simulink model "demo_interconnect"  (Simulink 7.4)
settings: Solver=ode45  StartTime=0.0  StopTime=100  RelTol=1e-3
undefined symbols (not defined in the file): ROACH
libraries: xbsIndex_r4 x135, xps_library x13, casper_library x12, isi_correlator_lib x10, dspsigops x8
settings Model: Creator=wjm  LastModifiedBy=wjm
settings OptimizationCC: InitFltsAndDblsToZero=on

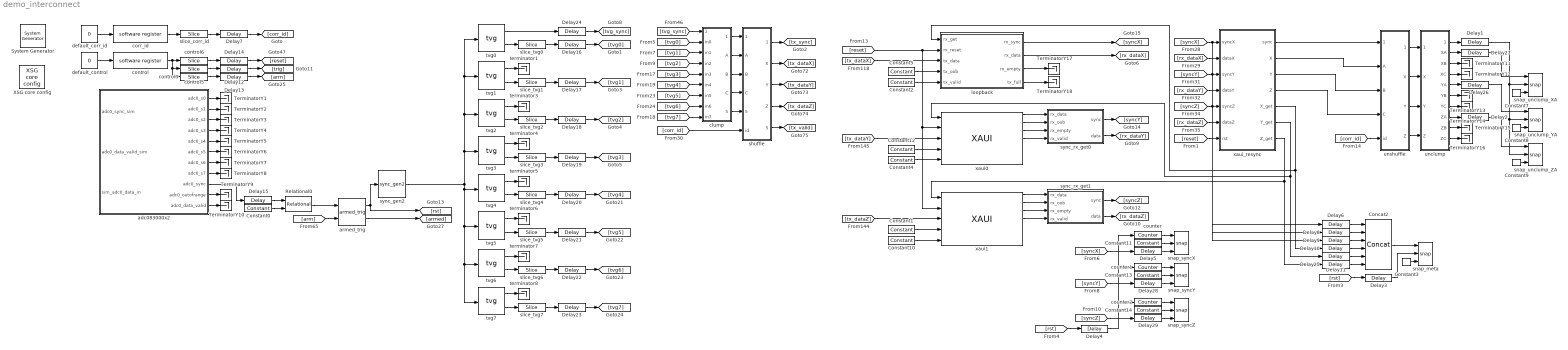
== system demo_interconnect ==
  " System Generator" : xbsIndex_r4/ System Generator  Tag=genX  SystemSampleTime=-1  xilinxfamily=virtex5  part=xc5vsx95t  speed=-1  package=ff1136  synthesis_tool=XST  clock_wrapper=Clock Enables  directory=./demo_interconnect/sysgen  testbench=off  simulink_period=1  sysclk_period=5  dcm_input_clock_period=100  incr_netlist=off  trim_vbits=Everywhere in SubSystem  dbl_ovrd=According to Block Masks  core_generation=According to Block Masks  run_coregen=off  deprecated_control=off  eval_field=0  block_type=sysgen
      settings: block_version=10.1.1
  Concat2 : xbsIndex_r4/Concat  num_inputs=6  dbl_ovrd=off  block_type=concat
      settings: block_version=11.3
  Constant{0..1,5,12} (4 alike) : xbsIndex_r4/Constant  arith_type=Unsigned  const=0  n_bits=4  bin_pt=0  explicit_period=on  period=1  equ=P=C  opselect=C  inp2=PCIN>>17  opr=+  inp1=P  carry=CIN  dbl_ovrd=off  block_type=constant
      Constant1 settings: block_version=10.1.1
      Constant12 settings: block_version=10.1.1
      Constant5 settings: block_version=10.1.1
  Constant{2..4,7..11,13..14} (10 alike) : xbsIndex_r4/Constant  arith_type=Boolean  const=1  n_bits=1  bin_pt=0  explicit_period=on  period=1  equ=P=C  opselect=C  inp2=PCIN>>17  opr=+  inp1=P  carry=CIN  dbl_ovrd=off  block_type=constant
      settings: block_version=10.1.1
  Delay{1..2,12..24,26..27} (17 alike) : xbsIndex_r4/Delay  en=off  latency=1  dbl_ovrd=off  reg_retiming=on  block_type=delay
  Delay{6,8..11,25} (6 alike) : xbsIndex_r4/Delay  en=off  latency=17  dbl_ovrd=off  reg_retiming=off  block_type=delay
  Delay{3..5,28..29} (5 alike) : xbsIndex_r4/Delay  en=off  latency=1  dbl_ovrd=off  reg_retiming=off  block_type=delay
  Delay7 : xbsIndex_r4/Delay  en=off  latency=0  dbl_ovrd=off  reg_retiming=on  block_type=delay
  Relational0 : xbsIndex_r4/Relational  mode=a!=b  en=off  latency=1  dbl_ovrd=off  block_type=relational
      settings: xl_area=[0, 0, 0, 0, 0, 0, 0]  block_version=10.1.3
  TerminatorY{1..18} (18 alike) : Terminator
  XSG core config : xps_library/XSG core config  Tag=xps:xsg  SystemSampleTime=-1  hw_sys=ROACH:sx95t  ibob_linux=off  clk_src=adc0_clk  iBOB_clk_src=sys_clk  BEE2_ctrl_clk_src=sys_clk  BEE2_usr_clk_src=sys_clk  ROACH_clk_src=adc0_clk  CORR_clk_src=sys_clk  gpio_clk_io_group=iBOB:sma  gpio_clk_bit_index=0  clk_rate=200  sample_period=1  synthesis_tool=XST  mpc_type=powerpc440_ext
  adc083000x2 : Subsystem  Tag=xps:adc083000x2  AncestorBlock=xps_library/adc083000x2  mask(adc_083000x2){use_adc0=on, use_adc1=off, demux_adc=off, clock_sync=off, verbose=off, using_ctrl=off, adc_clk_rate=800, sample_period=1, bit_width=8}
      mask prompts: use_adc0 "Use ZD0K0?"; use_adc1 "Use ZDOK1?"; demux_adc "Demux ADCs by 2?"; clock_sync "Interleave 2 ADC boards?"; verbose "Verbose Block Creation?"; using_ctrl "Add ports for control registers?"; adc_clk_rate "ADC clock rate (MHz)"; sample_period "Sample Period"; bit_width "Output Bit Width"
      mask help:
      | The ADC block converts analog inputs to digital outputs.
      | Every clock cycle, the inputs are sampled and digitized to
      | 8 bit binary point numbers in the range of [-1, 1).
      |
      | Online block-specific documentation: http://casper.berkeley.edu/wiki/Adc083000
      mask init:
      | adc083000_mask;
      mask Help: eval('xlWeb([getenv(''MLIB_ROOT''), ''\doc\html\sys_adc\sys_adc.html''])')
  armed_trig : isi_correlator_lib/armed_trig  SystemSampleTime=-1
  clump : Subsystem  AncestorBlock=isi_correlator_lib/clump  mask{latency=1}
  control : xps_library/software register  Tag=xps:sw_reg  SystemSampleTime=-1  io_dir=From Processor  arith_type=Unsigned  bitwidth=32  bin_pt=0  sample_period=1  gw_name=demo_interconnect_control_user_data_out
  control0 : xbsIndex_r4/Slice  nbits=1  boolean_output=on  mode=Lower Bit Location + Width  bit1=0  base1=MSB of Input  bit0=0  base0=LSB of Input  dbl_ovrd=off  block_type=slice
      settings: infoedit="Extracts a given range of bits from each input sample and presents it at the output.  The output type is ordinarily unsigned with binary point at zero, but can be Boolean when the slice is one bit wide.<P><P>Hardware notes: In hardware this block costs nothing."  block_version=10.1.3
  control5 : xbsIndex_r4/Slice  nbits=1  boolean_output=on  mode=Lower Bit Location + Width  bit1=0  base1=MSB of Input  bit0=1  base0=LSB of Input  dbl_ovrd=off  block_type=slice
      settings: infoedit="Extracts a given range of bits from each input sample and presents it at the output.  The output type is ordinarily unsigned with binary point at zero, but can be Boolean when the slice is one bit wide.<P><P>Hardware notes: In hardware this block costs nothing."  block_version=10.1.3
  control6 : xbsIndex_r4/Slice  nbits=1  boolean_output=on  mode=Lower Bit Location + Width  bit1=0  base1=MSB of Input  bit0=2  base0=LSB of Input  dbl_ovrd=off  block_type=slice
      settings: infoedit="Extracts a given range of bits from each input sample and presents it at the output.  The output type is ordinarily unsigned with binary point at zero, but can be Boolean when the slice is one bit wide.<P><P>Hardware notes: In hardware this block costs nothing."  block_version=10.1.3
  corr_id : xps_library/software register  Tag=xps:sw_reg  SystemSampleTime=-1  io_dir=From Processor  arith_type=Unsigned  bitwidth=32  bin_pt=0  sample_period=1  gw_name=demo_interconnect_corr_id_user_data_out
  counter : xbsIndex_r4/Counter  cnt_type=Free Running  cnt_to=Inf  operation=Up  start_count=0  cnt_by_val=1  arith_type=Unsigned  n_bits=32  bin_pt=0  load_pin=off  rst=on  en=off  explicit_period=on  period=1  dbl_ovrd=off  use_behavioral_HDL=off  implementation=Fabric  use_rpm=off  block_type=counter
  counter1 : xbsIndex_r4/Counter  cnt_type=Free Running  cnt_to=Inf  operation=Up  start_count=0  cnt_by_val=1  arith_type=Unsigned  n_bits=32  bin_pt=0  load_pin=off  rst=on  en=off  explicit_period=on  period=1  dbl_ovrd=off  use_behavioral_HDL=off  implementation=Fabric  use_rpm=off  block_type=counter
  counter2 : xbsIndex_r4/Counter  cnt_type=Free Running  cnt_to=Inf  operation=Up  start_count=0  cnt_by_val=1  arith_type=Unsigned  n_bits=32  bin_pt=0  load_pin=off  rst=on  en=off  explicit_period=on  period=1  dbl_ovrd=off  use_behavioral_HDL=off  implementation=Fabric  use_rpm=off  block_type=counter
  default_control : Constant  Value=0  OutDataType=sfix(16)  OutScaling=2^0  SampleTime=1
  default_corr_id : Constant  Value=0  OutDataType=sfix(16)  OutScaling=2^0  SampleTime=1
  loopback : Subsystem  AncestorBlock=isi_correlator_lib/loopback  mask(loopback){delay=8}
      mask prompts: delay "Delay: (2^?)"
      mask help:
      | A loopback link. Stores data in BRAM for long delay periods.
      |
      | Intended for buffering a stream of data until the other two
      | arrive over XAUI for resyncing.  Its delay should be set to
      | something on the order of (but less than) the XAUI latency.
  shuffle : Subsystem  AncestorBlock=isi_correlator_lib/shuffle  mask{latency=3}
  slice_corr_id : xbsIndex_r4/Slice  nbits=2  boolean_output=off  mode=Lower Bit Location + Width  bit1=0  base1=MSB of Input  bit0=0  base0=LSB of Input  dbl_ovrd=off  block_type=slice
      settings: infoedit="Extracts a given range of bits from each input sample and presents it at the output.  The output type is ordinarily unsigned with binary point at zero, but can be Boolean when the slice is one bit wide.<P><P>Hardware notes: In hardware this block costs nothing."  block_version=10.1.3
  slice_tvg{0..7} (8 alike) : xbsIndex_r4/Slice  nbits=8  boolean_output=off  mode=Lower Bit Location + Width  bit1=0  base1=MSB of Input  bit0=0  base0=LSB of Input  dbl_ovrd=off  block_type=slice
      settings: block_version=10.1.3
  snap_meta : casper_library/Scopes/snap  SystemSampleTime=-1  nsamples=13
  snap_syncX : casper_library/Scopes/snap  SystemSampleTime=-1  nsamples=13
  snap_syncY : casper_library/Scopes/snap  SystemSampleTime=-1  nsamples=13
  snap_syncZ : casper_library/Scopes/snap  SystemSampleTime=-1  nsamples=13
  snap_unclump_XA : casper_library/Scopes/snap  SystemSampleTime=-1  nsamples=13
  snap_unclump_YA : casper_library/Scopes/snap  SystemSampleTime=-1  nsamples=13
  snap_unclump_ZA : casper_library/Scopes/snap  SystemSampleTime=-1  nsamples=13
  sync_gen2 : isi_correlator_lib/sync_gen2  SystemSampleTime=-1
  sync_rx_get0 : Subsystem  AncestorBlock=isi_correlator_lib/sync_rx_get
  sync_rx_get1 : Subsystem  AncestorBlock=isi_correlator_lib/sync_rx_get
  terminator{1,3..8} (7 alike) : Terminator
  tvg{0..7} (8 alike) : isi_correlator_lib/tvg  SystemSampleTime=-1  addr_width=11
  unclump : Subsystem  AncestorBlock=isi_correlator_lib/unclump  mask{latency=1}
  unshuffle : Subsystem  AncestorBlock=isi_correlator_lib/unshuffle  mask{latency=3}
  xaui0 : xps_library/XAUI  Tag=xps:xaui  SystemSampleTime=-1  demux=2  port=ROACH:0  open_phy=off  show_param=off  pre_emph=3  swing=800
  xaui1 : xps_library/XAUI  Tag=xps:xaui  SystemSampleTime=-1  demux=2  port=ROACH:1  open_phy=off  show_param=off  pre_emph=3  swing=800
  xaui_resync : Subsystem  AncestorBlock=isi_correlator_lib/xaui_resync  mask(link_demux){buffer_depth=10, logic_latency=1}
      mask prompts: buffer_depth "Buffer depth: (2^?)"; logic_latency "Logic latency:"
      mask help:
      | Resynchronizes three data streams based on their sync pulses.
      |
      | Maximum buffer depth is 2^10.
  wires:
  armed_trig/1 -> sync_gen2/1, [rst]
  armed_trig/2 -> [armed]
  [tvg_sync] -> clump/1(sync)
  [tvg0] -> clump/2(in0)
  [tvg1] -> clump/3(in1)
  [tvg2] -> clump/4(in2)
  [tvg3] -> clump/5(in3)
  [tvg4] -> clump/6(in4)
  [tvg5] -> clump/7(in5)
  [tvg6] -> clump/8(in6)
  tvg0/2 -> slice_tvg0/1
  tvg1/2 -> slice_tvg1/1
  tvg2/2 -> slice_tvg2/1
  tvg0/1 -> Delay24/1
  tvg1/1 -> terminator1/1
  tvg2/1 -> terminator3/1
  tvg7/2 -> slice_tvg7/1
  tvg5/2 -> slice_tvg5/1
  tvg6/2 -> slice_tvg6/1
  tvg4/2 -> slice_tvg4/1
  tvg3/2 -> slice_tvg3/1
  tvg3/1 -> terminator4/1
  tvg4/1 -> terminator5/1
  tvg5/1 -> terminator6/1
  tvg6/1 -> terminator7/1
  tvg7/1 -> terminator8/1
  slice_tvg0/1 -> Delay16/1
  slice_tvg1/1 -> Delay17/1
  slice_tvg2/1 -> Delay18/1
  slice_tvg3/1 -> Delay19/1
  slice_tvg4/1 -> Delay20/1
  slice_tvg5/1 -> Delay21/1
  slice_tvg6/1 -> Delay22/1
  slice_tvg7/1 -> Delay23/1
  shuffle/1(sync_out) -> [tx_sync]
  shuffle/2(X) -> [tx_dataX]
  shuffle/3(Y) -> [tx_dataY]
  shuffle/4(Z) -> [tx_dataZ]
  shuffle/5(valid_out) -> [tx_valid]
  [tvg7] -> clump/9(in7)
  clump/1(sync_out) -> shuffle/1(sync)
  clump/2(A) -> shuffle/2(A)
  clump/3(B) -> shuffle/3(B)
  clump/4(C) -> shuffle/4(C)
  clump/5(valid) -> shuffle/5(valid)
  [corr_id] -> shuffle/6(id)
  unshuffle/1(sync_out) -> unclump/1(sync)
  unshuffle/2(X) -> unclump/2(X)
  unshuffle/3(Y) -> unclump/3(Y)
  unshuffle/4(Z) -> unclump/4(Z)
  [arm] -> armed_trig/2
  default_corr_id/1 -> corr_id/1
  corr_id/1 -> slice_corr_id/1
  Delay7/1 -> [corr_id]
  slice_corr_id/1 -> Delay7/1
  default_control/1 -> control/1
  control6/1 -> Delay14/1
  control5/1 -> Delay12/1
  control0/1 -> Delay13/1
  control/1 -> control6/1, control0/1, control5/1
  Delay14/1 -> [reset]
  Delay12/1 -> [trig]
  Delay13/1 -> [arm]
  adc083000x2/1(adc0_s0) -> TerminatorY1/1
  adc083000x2/2(adc0_s1) -> TerminatorY2/1
  adc083000x2/3(adc0_s2) -> TerminatorY3/1
  adc083000x2/4(adc0_s3) -> TerminatorY4/1
  adc083000x2/5(adc0_s4) -> TerminatorY5/1
  adc083000x2/6(adc0_s5) -> TerminatorY6/1
  adc083000x2/7(adc0_s6) -> TerminatorY7/1
  adc083000x2/8(adc0_s7) -> TerminatorY8/1
  adc083000x2/10(adc0_outofrange) -> TerminatorY9/1
  adc083000x2/11(adc0_data_valid) -> TerminatorY10/1
  Constant0/1 -> Relational0/2
  adc083000x2/9(adc0_sync) -> Delay15/1
  Delay15/1 -> Relational0/1
  Relational0/1 -> armed_trig/1
  sync_gen2/1 -> tvg4/1, tvg5/1, tvg7/1, tvg6/1, tvg3/1, tvg2/1, tvg0/1, tvg1/1
  Delay16/1 -> [tvg0]
  Delay17/1 -> [tvg1]
  Delay18/1 -> [tvg2]
  Delay19/1 -> [tvg3]
  Delay20/1 -> [tvg4]
  Delay21/1 -> [tvg5]
  Delay22/1 -> [tvg6]
  Delay23/1 -> [tvg7]
  Delay24/1 -> [tvg_sync]
  [tx_dataZ] -> xaui1/3
  Constant1/1 -> xaui1/4
  Constant12/1 -> xaui0/4
  [tx_dataY] -> xaui0/3
  Constant7/1 -> snap_unclump_XA/3
  Constant8/1 -> snap_unclump_YA/3
  Constant9/1 -> snap_unclump_ZA/3
  unclump/2(XA) -> Delay27/1
  unclump/5(YA) -> Delay26/1
  unclump/8(ZA) -> Delay2/1
  unclump/3(XB) -> TerminatorY11/1
  unclump/4(XC) -> TerminatorY12/1
  unclump/6(YB) -> TerminatorY13/1
  unclump/7(YC) -> TerminatorY14/1
  unclump/9(ZB) -> TerminatorY15/1
  unclump/10(ZC) -> TerminatorY16/1
  Delay2/1 -> snap_unclump_ZA/1
  Delay26/1 -> snap_unclump_YA/1
  Delay27/1 -> snap_unclump_XA/1
  xaui1/1 -> sync_rx_get1/1(rx_data)
  xaui1/2 -> sync_rx_get1/2(rx_oob)
  xaui1/3 -> sync_rx_get1/3(rx_empty)
  xaui1/4 -> sync_rx_get1/4(rx_valid)
  xaui0/1 -> sync_rx_get0/1(rx_data)
  xaui0/2 -> sync_rx_get0/2(rx_oob)
  xaui0/3 -> sync_rx_get0/3(rx_empty)
  xaui0/4 -> sync_rx_get0/4(rx_valid)
  [tx_dataX] -> loopback/3(tx_data)
  Constant2/1 -> loopback/5(tx_valid)
  Constant4/1 -> xaui0/5
  Constant10/1 -> xaui1/5
  [reset] -> loopback/2(rx_reset), xaui1/2, xaui0/2
  [corr_id] -> unshuffle/5(id)
  xaui_resync/1(sync) -> unshuffle/1(sync)
  xaui_resync/2(X) -> unshuffle/2(A)
  xaui_resync/3(Y) -> unshuffle/3(B)
  xaui_resync/4(Z) -> unshuffle/4(C)
  [syncX] -> xaui_resync/1(syncX), Delay6/1
  [rx_dataX] -> xaui_resync/2(dataX)
  [syncY] -> xaui_resync/3(syncY), Delay8/1
  [rx_dataY] -> xaui_resync/4(dataY)
  [syncZ] -> xaui_resync/5(syncZ), Delay9/1
  [rx_dataZ] -> xaui_resync/6(dataZ)
  xaui_resync/5(X_get) -> loopback/1(rx_get), Delay10/1
  xaui_resync/6(Y_get) -> xaui0/1, Delay11/1
  xaui_resync/7(Z_get) -> xaui1/1, Delay25/1
  [reset] -> xaui_resync/7(rst)
  loopback/1(rx_sync) -> [syncX]
  loopback/2(rx_data) -> [rx_dataX]
  Constant3/1 -> snap_meta/3
  Delay3/1 -> snap_meta/2
  [rst] -> Delay3/1
  Concat2/1 -> snap_meta/1
  sync_rx_get1/1(sync) -> [syncZ]
  sync_rx_get1/2(data) -> [rx_dataZ]
  sync_rx_get0/1(sync) -> [syncY]
  sync_rx_get0/2(data) -> [rx_dataY]
  Constant5/1 -> loopback/4(tx_oob)
  Delay6/1 -> Concat2/1
  Delay8/1 -> Concat2/2
  Delay9/1 -> Concat2/3
  Delay10/1 -> Concat2/4
  Delay11/1 -> Concat2/5
  Delay25/1 -> Concat2/6
  loopback/3(rx_empty) -> TerminatorY17/1
  loopback/4(tx_full) -> TerminatorY18/1
  Constant11/1 -> snap_syncX/2
  Constant13/1 -> snap_syncY/2
  Constant14/1 -> snap_syncZ/2
  [rst] -> Delay4/1
  counter/1 -> snap_syncX/1
  counter1/1 -> snap_syncY/1
  counter2/1 -> snap_syncZ/1
  Delay4/1 -> counter2/1, counter/1, counter1/1
  [syncX] -> Delay5/1
  [syncY] -> Delay28/1
  [syncZ] -> Delay29/1
  unclump/1(sync_out) -> Delay1/1
  Delay1/1 -> snap_unclump_XA/2, snap_unclump_ZA/2, snap_unclump_YA/2
  Delay5/1 -> snap_syncX/3
  Delay28/1 -> snap_syncY/3
  Delay29/1 -> snap_syncZ/3

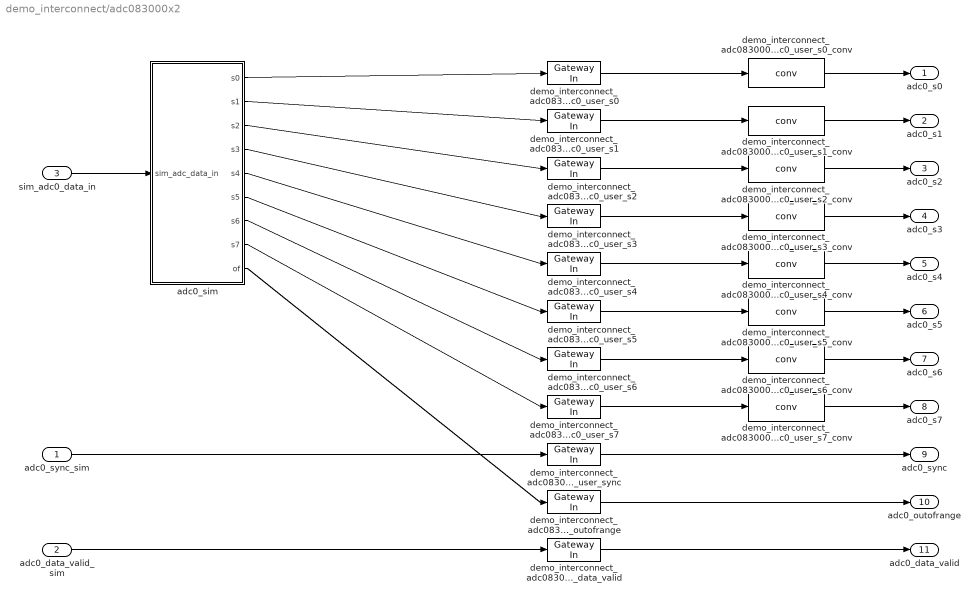
== system demo_interconnect/adc083000x2 ==
  adc0_sync_sim : Inport  OutDataType=sfix(16)  OutScaling=2^0
  adc0_data_valid_sim : Inport  Port=2  OutDataType=sfix(16)  OutScaling=2^0
  sim_adc0_data_in : Inport  Port=3  OutDataType=fixdt(1, 16)  OutScaling=2^0
  adc0_sim : Subsystem  AncestorBlock=xps_library/ADCs/adc_sim  mask(adc_sim){nStreams=8, bit_width=8}
      mask prompts: nStreams "Number of Output Streams"; bit_width "Sample Bit Width"
      mask help:
      | This block simulates the behavior of a demuxed ADC, which takes
      | as input a waveform and returns digital samples in parallel at
      | a slower rate.
      |
      | This block is used to simulate the behavior
      mask init:
      | adc_sim_init(gcb, ...
      |     'nStreams', nStreams, ...
      |     'bit_width', bit_width);
  demo_interconnect_adc083000x2_adc0_user_data_valid : xbsIndex_r4/Gateway In  arith_type=Unsigned  n_bits=1  bin_pt=0  quantization="Round  (unbiased: +/- Inf)"  overflow=Saturate  period=1  dbl_ovrd=off  timing_constraint=None  locs_specified=off  LOCs={}  hdl_port=on  block_type=gatewayin
      settings: infoedit="Gateway in block.  Converts inputs of type Simulink integer, double and fixed point to  Xilinx fixed point type.<br><br>Hardware notes:  In hardware these blocks become top level input ports."  block_version=11.4
  demo_interconnect_adc083000x2_adc0_user_outofrange : xbsIndex_r4/Gateway In  arith_type=Unsigned  n_bits=4  bin_pt=0  quantization="Round  (unbiased: +/- Inf)"  overflow=Saturate  period=1  dbl_ovrd=off  timing_constraint=None  locs_specified=off  LOCs={}  hdl_port=on  block_type=gatewayin
      settings: infoedit="Gateway in block.  Converts inputs of type Simulink integer, double and fixed point to  Xilinx fixed point type.<br><br>Hardware notes:  In hardware these blocks become top level input ports."  block_version=11.4
  demo_interconnect_adc083000x2_adc0_user_s{0..7} (8 alike) : xbsIndex_r4/Gateway In  arith_type=Unsigned  n_bits=8  bin_pt=0  quantization="Round  (unbiased: +/- Inf)"  overflow=Saturate  period=1  dbl_ovrd=off  timing_constraint=None  locs_specified=off  LOCs={}  hdl_port=on  block_type=gatewayin
      settings: infoedit="Gateway in block.  Converts inputs of type Simulink integer, double and fixed point to  Xilinx fixed point type.<br><br>Hardware notes:  In hardware these blocks become top level input ports."  block_version=11.4
  demo_interconnect_adc083000x2_adc0_user_s0_conv : xps_library/ADCs/conv  SystemSampleTime=-1  bit_width=8
  demo_interconnect_adc083000x2_adc0_user_s1_conv : xps_library/ADCs/conv  SystemSampleTime=-1  bit_width=8
  demo_interconnect_adc083000x2_adc0_user_s2_conv : xps_library/ADCs/conv  SystemSampleTime=-1  bit_width=8
  demo_interconnect_adc083000x2_adc0_user_s3_conv : xps_library/ADCs/conv  SystemSampleTime=-1  bit_width=8
  demo_interconnect_adc083000x2_adc0_user_s4_conv : xps_library/ADCs/conv  SystemSampleTime=-1  bit_width=8
  demo_interconnect_adc083000x2_adc0_user_s5_conv : xps_library/ADCs/conv  SystemSampleTime=-1  bit_width=8
  demo_interconnect_adc083000x2_adc0_user_s6_conv : xps_library/ADCs/conv  SystemSampleTime=-1  bit_width=8
  demo_interconnect_adc083000x2_adc0_user_s7_conv : xps_library/ADCs/conv  SystemSampleTime=-1  bit_width=8
  demo_interconnect_adc083000x2_adc0_user_sync : xbsIndex_r4/Gateway In  arith_type=Unsigned  n_bits=4  bin_pt=0  quantization="Round  (unbiased: +/- Inf)"  overflow=Saturate  period=1  dbl_ovrd=off  timing_constraint=None  locs_specified=off  LOCs={}  hdl_port=on  block_type=gatewayin
      settings: infoedit="Gateway in block.  Converts inputs of type Simulink integer, double and fixed point to  Xilinx fixed point type.<br><br>Hardware notes:  In hardware these blocks become top level input ports."  block_version=11.4
  adc0_s0 : Outport  OutDataType=fixdt(1, 16)  OutScaling=2^0
  adc0_s1 : Outport  Port=2  OutDataType=fixdt(1, 16)  OutScaling=2^0
  adc0_s2 : Outport  Port=3  OutDataType=fixdt(1, 16)  OutScaling=2^0
  adc0_s3 : Outport  Port=4  OutDataType=fixdt(1, 16)  OutScaling=2^0
  adc0_s4 : Outport  Port=5  OutDataType=fixdt(1, 16)  OutScaling=2^0
  adc0_s5 : Outport  Port=6  OutDataType=fixdt(1, 16)  OutScaling=2^0
  adc0_s6 : Outport  Port=7  OutDataType=fixdt(1, 16)  OutScaling=2^0
  adc0_s7 : Outport  Port=8  OutDataType=fixdt(1, 16)  OutScaling=2^0
  adc0_sync : Outport  Port=9  OutDataType=sfix(16)  OutScaling=2^0
  adc0_outofrange : Outport  Port=10  OutDataType=fixdt(1, 16)  OutScaling=2^0
  adc0_data_valid : Outport  Port=11  OutDataType=sfix(16)  OutScaling=2^0
  wires:
  sim_adc0_data_in/1 -> adc0_sim/1(sim_adc_data_in)
  adc0_sim/1(s0) -> demo_interconnect_adc083000x2_adc0_user_s0/1
  demo_interconnect_adc083000x2_adc0_user_s0/1 -> demo_interconnect_adc083000x2_adc0_user_s0_conv/1
  demo_interconnect_adc083000x2_adc0_user_s0_conv/1 -> adc0_s0/1
  adc0_sim/2(s1) -> demo_interconnect_adc083000x2_adc0_user_s1/1
  demo_interconnect_adc083000x2_adc0_user_s1/1 -> demo_interconnect_adc083000x2_adc0_user_s1_conv/1
  demo_interconnect_adc083000x2_adc0_user_s1_conv/1 -> adc0_s1/1
  adc0_sim/3(s2) -> demo_interconnect_adc083000x2_adc0_user_s2/1
  demo_interconnect_adc083000x2_adc0_user_s2/1 -> demo_interconnect_adc083000x2_adc0_user_s2_conv/1
  demo_interconnect_adc083000x2_adc0_user_s2_conv/1 -> adc0_s2/1
  adc0_sim/4(s3) -> demo_interconnect_adc083000x2_adc0_user_s3/1
  demo_interconnect_adc083000x2_adc0_user_s3/1 -> demo_interconnect_adc083000x2_adc0_user_s3_conv/1
  demo_interconnect_adc083000x2_adc0_user_s3_conv/1 -> adc0_s3/1
  adc0_sim/5(s4) -> demo_interconnect_adc083000x2_adc0_user_s4/1
  demo_interconnect_adc083000x2_adc0_user_s4/1 -> demo_interconnect_adc083000x2_adc0_user_s4_conv/1
  demo_interconnect_adc083000x2_adc0_user_s4_conv/1 -> adc0_s4/1
  adc0_sim/6(s5) -> demo_interconnect_adc083000x2_adc0_user_s5/1
  demo_interconnect_adc083000x2_adc0_user_s5/1 -> demo_interconnect_adc083000x2_adc0_user_s5_conv/1
  demo_interconnect_adc083000x2_adc0_user_s5_conv/1 -> adc0_s5/1
  adc0_sim/7(s6) -> demo_interconnect_adc083000x2_adc0_user_s6/1
  demo_interconnect_adc083000x2_adc0_user_s6/1 -> demo_interconnect_adc083000x2_adc0_user_s6_conv/1
  demo_interconnect_adc083000x2_adc0_user_s6_conv/1 -> adc0_s6/1
  adc0_sim/8(s7) -> demo_interconnect_adc083000x2_adc0_user_s7/1
  demo_interconnect_adc083000x2_adc0_user_s7/1 -> demo_interconnect_adc083000x2_adc0_user_s7_conv/1
  demo_interconnect_adc083000x2_adc0_user_s7_conv/1 -> adc0_s7/1
  adc0_sync_sim/1 -> demo_interconnect_adc083000x2_adc0_user_sync/1
  demo_interconnect_adc083000x2_adc0_user_sync/1 -> adc0_sync/1
  adc0_sim/9(of) -> demo_interconnect_adc083000x2_adc0_user_outofrange/1
  demo_interconnect_adc083000x2_adc0_user_outofrange/1 -> adc0_outofrange/1
  adc0_data_valid_sim/1 -> demo_interconnect_adc083000x2_adc0_user_data_valid/1
  demo_interconnect_adc083000x2_adc0_user_data_valid/1 -> adc0_data_valid/1

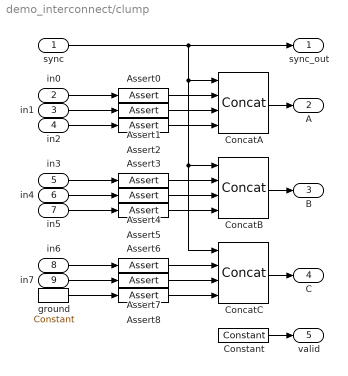
== system demo_interconnect/clump ==
  sync : Inport
  in0 : Inport  Port=2
  in1 : Inport  Port=3
  in2 : Inport  Port=4
  in3 : Inport  Port=5
  in4 : Inport  Port=6
  in5 : Inport  Port=7
  in6 : Inport  Port=8
  in7 : Inport  Port=9
  Assert{0..8} (9 alike) : xbsIndex_r4/Assert  assert_type=on  type_source=Explicitly  arith_type=Unsigned  n_bits=8  bin_pt=0  assert_rate=on  rate_source=Explicitly  period=1  output_port=on  block_type=assert
      settings: block_version=11.4
  ConcatA : xbsIndex_r4/Concat  num_inputs=4  dbl_ovrd=off  block_type=concat
      settings: block_version=11.3
  ConcatB : xbsIndex_r4/Concat  num_inputs=4  dbl_ovrd=off  block_type=concat
      settings: block_version=11.3
  ConcatC : xbsIndex_r4/Concat  num_inputs=4  dbl_ovrd=off  block_type=concat
      settings: block_version=11.3
  Constant : xbsIndex_r4/Constant  arith_type=Boolean  const=1  n_bits=1  bin_pt=0  explicit_period=on  period=1  equ=P=C  opselect=C  inp2=PCIN>>17  opr=+  inp1=P  carry=CIN  dbl_ovrd=off  block_type=constant
      settings: block_version=11.4
  ground : xbsIndex_r4/Constant  arith_type=Unsigned  const=0  n_bits=8  bin_pt=0  explicit_period=on  period=1  equ=P=C  opselect=C  inp2=PCIN>>17  opr=+  inp1=P  carry=CIN  dbl_ovrd=off  block_type=constant
      settings: block_version=10.1.1
  sync_out : Outport
  A : Outport  Port=2
  B : Outport  Port=3
  C : Outport  Port=4
  valid : Outport  Port=5
  wires:
  in2/1 -> Assert2/1
  in1/1 -> Assert1/1
  in0/1 -> Assert0/1
  ground/1 -> Assert8/1
  in7/1 -> Assert7/1
  in6/1 -> Assert6/1
  in5/1 -> Assert5/1
  in4/1 -> Assert4/1
  in3/1 -> Assert3/1
  sync/1 -> sync_out/1, ConcatA/1, ConcatC/1, ConcatB/1
  Constant/1 -> valid/1
  ConcatA/1 -> A/1
  ConcatB/1 -> B/1
  ConcatC/1 -> C/1
  Assert0/1 -> ConcatA/2
  Assert1/1 -> ConcatA/3
  Assert2/1 -> ConcatA/4
  Assert3/1 -> ConcatB/2
  Assert4/1 -> ConcatB/3
  Assert5/1 -> ConcatB/4
  Assert6/1 -> ConcatC/2
  Assert7/1 -> ConcatC/3
  Assert8/1 -> ConcatC/4

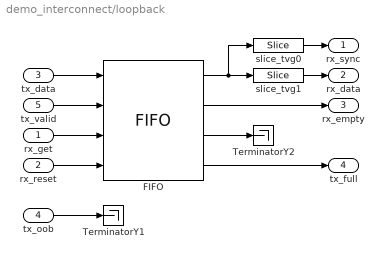
== system demo_interconnect/loopback ==
  rx_get : Inport  OutDataType=sfix(16)  OutScaling=2^0
  rx_reset : Inport  Port=2  OutDataType=sfix(16)  OutScaling=2^0
  tx_data : Inport  Port=3  OutDataType=sfix(16)  OutScaling=2^0
  tx_oob : Inport  Port=4  OutDataType=sfix(16)  OutScaling=2^0
  tx_valid : Inport  Port=5  OutDataType=sfix(16)  OutScaling=2^0
  FIFO : xbsIndex_r4/FIFO  depth=4K  percent_nbits=1  rst=on  en=off  use_dcount=off  use_almost_empty=off  almost_empty_thresh=2  use_almost_full=off  almost_full_thresh=14  dbl_ovrd=off  mem_type=Block RAM  explicit_period=off  block_type=fifo
      settings: block_version=11.4
  TerminatorY1 : Terminator
  TerminatorY2 : Terminator
  slice_tvg0 : xbsIndex_r4/Slice  nbits=1  boolean_output=on  mode=Lower Bit Location + Width  bit1=0  base1=MSB of Input  bit0=24  base0=LSB of Input  dbl_ovrd=off  block_type=slice
      settings: block_version=10.1.3
  slice_tvg1 : xbsIndex_r4/Slice  nbits=24  boolean_output=off  mode=Lower Bit Location + Width  bit1=0  base1=MSB of Input  bit0=0  base0=LSB of Input  dbl_ovrd=off  block_type=slice
      settings: block_version=10.1.3
  rx_sync : Outport  OutDataType=sfix(16)  OutScaling=2^0
  rx_data : Outport  Port=2  OutDataType=sfix(16)  OutScaling=2^0
  rx_empty : Outport  Port=3  OutDataType=sfix(16)  OutScaling=2^0
  tx_full : Outport  Port=4  OutDataType=sfix(16)  OutScaling=2^0
  wires:
  tx_data/1 -> FIFO/1
  tx_valid/1 -> FIFO/2
  rx_get/1 -> FIFO/3
  rx_reset/1 -> FIFO/4
  FIFO/2 -> rx_empty/1
  FIFO/1 -> slice_tvg1/1, slice_tvg0/1
  tx_oob/1 -> TerminatorY1/1
  slice_tvg1/1 -> rx_data/1
  slice_tvg0/1 -> rx_sync/1
  FIFO/4 -> tx_full/1
  FIFO/3 -> TerminatorY2/1

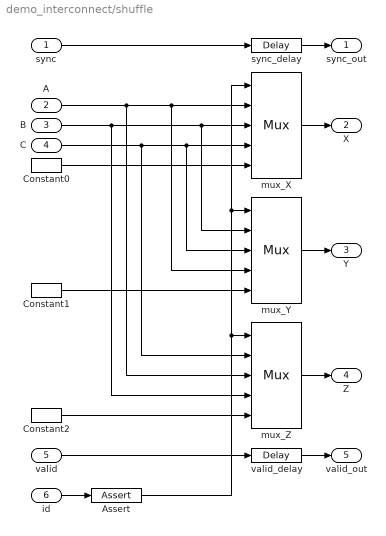
== system demo_interconnect/shuffle ==
  sync : Inport  OutDataType=sfix(16)  OutScaling=2^0
  A : Inport  Port=2  OutDataType=sfix(16)  OutScaling=2^0
  B : Inport  Port=3  OutDataType=sfix(16)  OutScaling=2^0
  C : Inport  Port=4  OutDataType=sfix(16)  OutScaling=2^0
  valid : Inport  Port=5  OutDataType=sfix(16)  OutScaling=2^0
  id : Inport  Port=6  OutDataType=sfix(16)  OutScaling=2^0
  Assert : xbsIndex_r4/Assert  assert_type=on  type_source=Explicitly  arith_type=Unsigned  n_bits=2  bin_pt=0  assert_rate=on  rate_source=Explicitly  period=1  output_port=on  block_type=assert
      settings: block_version=11.4
  Constant0 : xbsIndex_r4/Constant  arith_type=Unsigned  const=0  n_bits=25  bin_pt=0  explicit_period=on  period=1  equ=P=C  opselect=C  inp2=PCIN>>17  opr=+  inp1=P  carry=CIN  dbl_ovrd=off  block_type=constant
      settings: block_version=10.1.1
  Constant1 : xbsIndex_r4/Constant  arith_type=Unsigned  const=0  n_bits=25  bin_pt=0  explicit_period=on  period=1  equ=P=C  opselect=C  inp2=PCIN>>17  opr=+  inp1=P  carry=CIN  dbl_ovrd=off  block_type=constant
      settings: block_version=10.1.1
  Constant2 : xbsIndex_r4/Constant  arith_type=Unsigned  const=0  n_bits=25  bin_pt=0  explicit_period=on  period=1  equ=P=C  opselect=C  inp2=PCIN>>17  opr=+  inp1=P  carry=CIN  dbl_ovrd=off  block_type=constant
      settings: block_version=10.1.1
  mux_X : xbsIndex_r4/Mux  inputs=4  en=off  latency=latency  precision=Full  arith_type=Unsigned  n_bits=16  bin_pt=14  quantization=Truncate  overflow=Wrap  dbl_ovrd=off  block_type=mux
  mux_Y : xbsIndex_r4/Mux  inputs=4  en=off  latency=latency  precision=Full  arith_type=Unsigned  n_bits=16  bin_pt=14  quantization=Truncate  overflow=Wrap  dbl_ovrd=off  block_type=mux
  mux_Z : xbsIndex_r4/Mux  inputs=4  en=off  latency=latency  precision=Full  arith_type=Unsigned  n_bits=16  bin_pt=14  quantization=Truncate  overflow=Wrap  dbl_ovrd=off  block_type=mux
  sync_delay : xbsIndex_r4/Delay  en=off  latency=latency  dbl_ovrd=off  reg_retiming=off  block_type=delay
  valid_delay : xbsIndex_r4/Delay  en=off  latency=latency  dbl_ovrd=off  reg_retiming=off  block_type=delay
  sync_out : Outport  OutDataType=sfix(16)  OutScaling=2^0
  X : Outport  Port=2  OutDataType=sfix(16)  OutScaling=2^0
  Y : Outport  Port=3  OutDataType=sfix(16)  OutScaling=2^0
  Z : Outport  Port=4  OutDataType=sfix(16)  OutScaling=2^0
  valid_out : Outport  Port=5  OutDataType=sfix(16)  OutScaling=2^0
  wires:
  valid_delay/1 -> valid_out/1
  valid/1 -> valid_delay/1
  Assert/1 -> mux_Z/1, mux_Y/1, mux_X/1
  mux_Z/1 -> Z/1
  sync_delay/1 -> sync_out/1
  id/1 -> Assert/1
  sync/1 -> sync_delay/1
  C/1 -> mux_Z/2, mux_Y/3, mux_X/4
  B/1 -> mux_Z/4, mux_Y/2, mux_X/3
  A/1 -> mux_Z/3, mux_Y/4, mux_X/2
  mux_Y/1 -> Y/1
  mux_X/1 -> X/1
  Constant0/1 -> mux_X/5
  Constant1/1 -> mux_Y/5
  Constant2/1 -> mux_Z/5

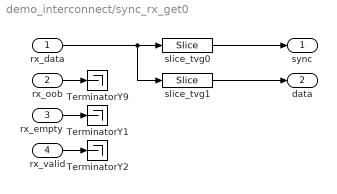
== system demo_interconnect/sync_rx_get0 ==
  rx_data : Inport
  rx_oob : Inport  Port=2
  rx_empty : Inport  Port=3
  rx_valid : Inport  Port=4
  TerminatorY1 : Terminator
  TerminatorY2 : Terminator
  TerminatorY9 : Terminator
  slice_tvg0 : xbsIndex_r4/Slice  nbits=1  boolean_output=on  mode=Lower Bit Location + Width  bit1=0  base1=MSB of Input  bit0=24  base0=LSB of Input  dbl_ovrd=off  block_type=slice
      settings: block_version=10.1.3
  slice_tvg1 : xbsIndex_r4/Slice  nbits=24  boolean_output=off  mode=Lower Bit Location + Width  bit1=0  base1=MSB of Input  bit0=0  base0=LSB of Input  dbl_ovrd=off  block_type=slice
      settings: block_version=10.1.3
  sync : Outport
  data : Outport  Port=2
  wires:
  rx_data/1 -> slice_tvg0/1, slice_tvg1/1
  slice_tvg0/1 -> sync/1
  slice_tvg1/1 -> data/1
  rx_oob/1 -> TerminatorY9/1
  rx_empty/1 -> TerminatorY1/1
  rx_valid/1 -> TerminatorY2/1

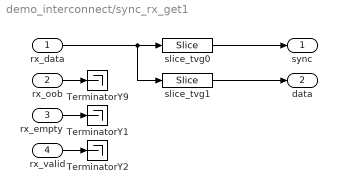
== system demo_interconnect/sync_rx_get1 ==
  rx_data : Inport
  rx_oob : Inport  Port=2
  rx_empty : Inport  Port=3
  rx_valid : Inport  Port=4
  TerminatorY1 : Terminator
  TerminatorY2 : Terminator
  TerminatorY9 : Terminator
  slice_tvg0 : xbsIndex_r4/Slice  nbits=1  boolean_output=on  mode=Lower Bit Location + Width  bit1=0  base1=MSB of Input  bit0=24  base0=LSB of Input  dbl_ovrd=off  block_type=slice
      settings: block_version=10.1.3
  slice_tvg1 : xbsIndex_r4/Slice  nbits=24  boolean_output=off  mode=Lower Bit Location + Width  bit1=0  base1=MSB of Input  bit0=0  base0=LSB of Input  dbl_ovrd=off  block_type=slice
      settings: block_version=10.1.3
  sync : Outport
  data : Outport  Port=2
  wires:
  rx_valid/1 -> TerminatorY2/1
  rx_empty/1 -> TerminatorY1/1
  rx_oob/1 -> TerminatorY9/1
  slice_tvg1/1 -> data/1
  slice_tvg0/1 -> sync/1
  rx_data/1 -> slice_tvg1/1, slice_tvg0/1

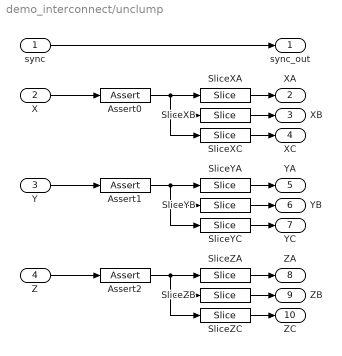
== system demo_interconnect/unclump ==
  sync : Inport
  X : Inport  Port=2
  Y : Inport  Port=3
  Z : Inport  Port=4
  Assert0 : xbsIndex_r4/Assert  assert_type=on  type_source=Explicitly  arith_type=Unsigned  n_bits=24  bin_pt=0  assert_rate=on  rate_source=Explicitly  period=1  output_port=on  block_type=assert
      settings: block_version=11.4
  Assert1 : xbsIndex_r4/Assert  assert_type=on  type_source=Explicitly  arith_type=Unsigned  n_bits=24  bin_pt=0  assert_rate=on  rate_source=Explicitly  period=1  output_port=on  block_type=assert
      settings: block_version=11.4
  Assert2 : xbsIndex_r4/Assert  assert_type=on  type_source=Explicitly  arith_type=Unsigned  n_bits=24  bin_pt=0  assert_rate=on  rate_source=Explicitly  period=1  output_port=on  block_type=assert
      settings: block_version=11.4
  SliceXA : xbsIndex_r4/Slice  nbits=8  boolean_output=off  mode=Lower Bit Location + Width  bit1=0  base1=MSB of Input  bit0=16  base0=LSB of Input  dbl_ovrd=off  block_type=slice
      settings: block_version=10.1.1
  SliceXB : xbsIndex_r4/Slice  nbits=8  boolean_output=off  mode=Lower Bit Location + Width  bit1=0  base1=MSB of Input  bit0=8  base0=LSB of Input  dbl_ovrd=off  block_type=slice
      settings: block_version=10.1.1
  SliceXC : xbsIndex_r4/Slice  nbits=8  boolean_output=off  mode=Lower Bit Location + Width  bit1=0  base1=MSB of Input  bit0=0  base0=LSB of Input  dbl_ovrd=off  block_type=slice
      settings: block_version=10.1.1
  SliceYA : xbsIndex_r4/Slice  nbits=8  boolean_output=off  mode=Lower Bit Location + Width  bit1=0  base1=MSB of Input  bit0=16  base0=LSB of Input  dbl_ovrd=off  block_type=slice
      settings: block_version=10.1.1
  SliceYB : xbsIndex_r4/Slice  nbits=8  boolean_output=off  mode=Lower Bit Location + Width  bit1=0  base1=MSB of Input  bit0=8  base0=LSB of Input  dbl_ovrd=off  block_type=slice
      settings: block_version=10.1.1
  SliceYC : xbsIndex_r4/Slice  nbits=8  boolean_output=off  mode=Lower Bit Location + Width  bit1=0  base1=MSB of Input  bit0=0  base0=LSB of Input  dbl_ovrd=off  block_type=slice
      settings: block_version=10.1.1
  SliceZA : xbsIndex_r4/Slice  nbits=8  boolean_output=off  mode=Lower Bit Location + Width  bit1=0  base1=MSB of Input  bit0=16  base0=LSB of Input  dbl_ovrd=off  block_type=slice
      settings: block_version=10.1.1
  SliceZB : xbsIndex_r4/Slice  nbits=8  boolean_output=off  mode=Lower Bit Location + Width  bit1=0  base1=MSB of Input  bit0=8  base0=LSB of Input  dbl_ovrd=off  block_type=slice
      settings: block_version=10.1.1
  SliceZC : xbsIndex_r4/Slice  nbits=8  boolean_output=off  mode=Lower Bit Location + Width  bit1=0  base1=MSB of Input  bit0=0  base0=LSB of Input  dbl_ovrd=off  block_type=slice
      settings: block_version=10.1.1
  sync_out : Outport
  XA : Outport  Port=2
  XB : Outport  Port=3
  XC : Outport  Port=4
  YA : Outport  Port=5
  YB : Outport  Port=6
  YC : Outport  Port=7
  ZA : Outport  Port=8
  ZB : Outport  Port=9
  ZC : Outport  Port=10
  wires:
  sync/1 -> sync_out/1
  X/1 -> Assert0/1
  Y/1 -> Assert1/1
  Z/1 -> Assert2/1
  Assert0/1 -> SliceXA/1, SliceXC/1, SliceXB/1
  Assert1/1 -> SliceYA/1, SliceYC/1, SliceYB/1
  Assert2/1 -> SliceZA/1, SliceZC/1, SliceZB/1
  SliceXA/1 -> XA/1
  SliceXB/1 -> XB/1
  SliceXC/1 -> XC/1
  SliceYA/1 -> YA/1
  SliceYB/1 -> YB/1
  SliceYC/1 -> YC/1
  SliceZA/1 -> ZA/1
  SliceZB/1 -> ZB/1
  SliceZC/1 -> ZC/1

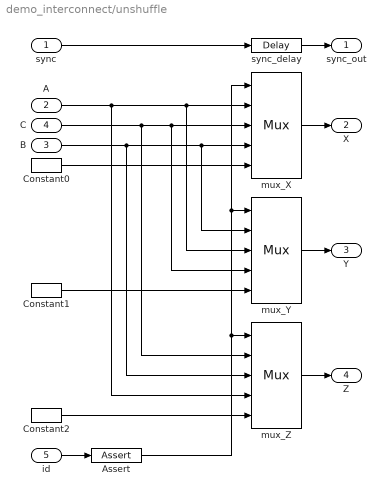
== system demo_interconnect/unshuffle ==
  sync : Inport  OutDataType=sfix(16)  OutScaling=2^0
  A : Inport  Port=2  OutDataType=sfix(16)  OutScaling=2^0
  B : Inport  Port=3  OutDataType=sfix(16)  OutScaling=2^0
  C : Inport  Port=4  OutDataType=sfix(16)  OutScaling=2^0
  id : Inport  Port=5  OutDataType=sfix(16)  OutScaling=2^0
  Assert : xbsIndex_r4/Assert  assert_type=on  type_source=Explicitly  arith_type=Unsigned  n_bits=2  bin_pt=0  assert_rate=on  rate_source=Explicitly  period=1  output_port=on  block_type=assert
      settings: block_version=11.4
  Constant0 : xbsIndex_r4/Constant  arith_type=Unsigned  const=0  n_bits=24  bin_pt=0  explicit_period=on  period=1  equ=P=C  opselect=C  inp2=PCIN>>17  opr=+  inp1=P  carry=CIN  dbl_ovrd=off  block_type=constant
      settings: block_version=10.1.1
  Constant1 : xbsIndex_r4/Constant  arith_type=Unsigned  const=0  n_bits=24  bin_pt=0  explicit_period=on  period=1  equ=P=C  opselect=C  inp2=PCIN>>17  opr=+  inp1=P  carry=CIN  dbl_ovrd=off  block_type=constant
      settings: block_version=10.1.1
  Constant2 : xbsIndex_r4/Constant  arith_type=Unsigned  const=0  n_bits=24  bin_pt=0  explicit_period=on  period=1  equ=P=C  opselect=C  inp2=PCIN>>17  opr=+  inp1=P  carry=CIN  dbl_ovrd=off  block_type=constant
      settings: block_version=10.1.1
  mux_X : xbsIndex_r4/Mux  inputs=4  en=off  latency=latency  precision=Full  arith_type=Unsigned  n_bits=16  bin_pt=14  quantization=Truncate  overflow=Wrap  dbl_ovrd=off  block_type=mux
  mux_Y : xbsIndex_r4/Mux  inputs=4  en=off  latency=latency  precision=Full  arith_type=Unsigned  n_bits=16  bin_pt=14  quantization=Truncate  overflow=Wrap  dbl_ovrd=off  block_type=mux
  mux_Z : xbsIndex_r4/Mux  inputs=4  en=off  latency=latency  precision=Full  arith_type=Unsigned  n_bits=16  bin_pt=14  quantization=Truncate  overflow=Wrap  dbl_ovrd=off  block_type=mux
  sync_delay : xbsIndex_r4/Delay  en=off  latency=latency  dbl_ovrd=off  reg_retiming=off  block_type=delay
  sync_out : Outport  OutDataType=sfix(16)  OutScaling=2^0
  X : Outport  Port=2  OutDataType=sfix(16)  OutScaling=2^0
  Y : Outport  Port=3  OutDataType=sfix(16)  OutScaling=2^0
  Z : Outport  Port=4  OutDataType=sfix(16)  OutScaling=2^0
  wires:
  Constant2/1 -> mux_Z/5
  Constant1/1 -> mux_Y/5
  Constant0/1 -> mux_X/5
  mux_X/1 -> X/1
  mux_Y/1 -> Y/1
  A/1 -> mux_Z/4, mux_X/2, mux_Y/3
  C/1 -> mux_X/3, mux_Y/4, mux_Z/2
  B/1 -> mux_X/4, mux_Y/2, mux_Z/3
  sync/1 -> sync_delay/1
  id/1 -> Assert/1
  sync_delay/1 -> sync_out/1
  mux_Z/1 -> Z/1
  Assert/1 -> mux_X/1, mux_Y/1, mux_Z/1

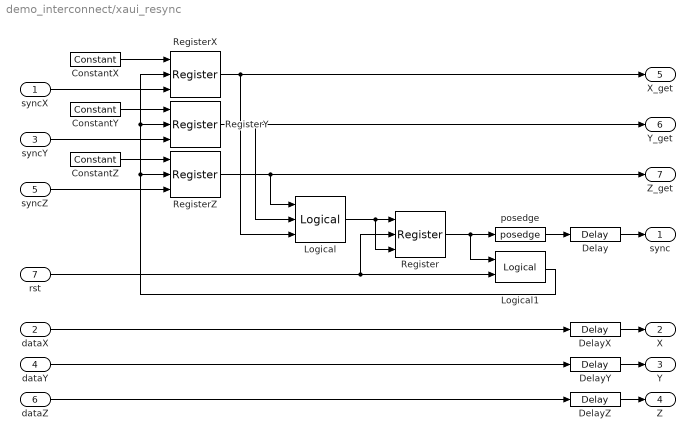
== system demo_interconnect/xaui_resync ==
  syncX : Inport  OutDataType=sfix(16)  OutScaling=2^0
  dataX : Inport  Port=2  OutDataType=sfix(16)  OutScaling=2^0
  syncY : Inport  Port=3  OutDataType=sfix(16)  OutScaling=2^0
  dataY : Inport  Port=4  OutDataType=sfix(16)  OutScaling=2^0
  syncZ : Inport  Port=5  OutDataType=sfix(16)  OutScaling=2^0
  dataZ : Inport  Port=6  OutDataType=sfix(16)  OutScaling=2^0
  rst : Inport  Port=7  OutDataType=sfix(16)  OutScaling=2^0
  ConstantX : xbsIndex_r4/Constant  arith_type=Boolean  const=0  n_bits=1  bin_pt=0  explicit_period=on  period=1  equ=P=C  opselect=C  inp2=PCIN>>17  opr=+  inp1=P  carry=CIN  dbl_ovrd=off  block_type=constant
      settings: block_version=10.1.1
  ConstantY : xbsIndex_r4/Constant  arith_type=Boolean  const=0  n_bits=1  bin_pt=0  explicit_period=on  period=1  equ=P=C  opselect=C  inp2=PCIN>>17  opr=+  inp1=P  carry=CIN  dbl_ovrd=off  block_type=constant
      settings: block_version=10.1.1
  ConstantZ : xbsIndex_r4/Constant  arith_type=Boolean  const=0  n_bits=1  bin_pt=0  explicit_period=on  period=1  equ=P=C  opselect=C  inp2=PCIN>>17  opr=+  inp1=P  carry=CIN  dbl_ovrd=off  block_type=constant
      settings: block_version=10.1.1
  Delay : xbsIndex_r4/Delay  en=off  latency=1  dbl_ovrd=off  reg_retiming=on  block_type=delay
  DelayX : xbsIndex_r4/Delay  en=off  latency=1  dbl_ovrd=off  reg_retiming=on  block_type=delay
  DelayY : xbsIndex_r4/Delay  en=off  latency=logic_latency  dbl_ovrd=off  reg_retiming=on  block_type=delay
  DelayZ : xbsIndex_r4/Delay  en=off  latency=logic_latency  dbl_ovrd=off  reg_retiming=on  block_type=delay
  Logical : xbsIndex_r4/Logical  logical_function=NOR  inputs=3  en=off  latency=1  precision=Full  arith_type=Unsigned  n_bits=16  bin_pt=0  align_bp=on  dbl_ovrd=off  block_type=logical
      settings: block_version=11.4
  Logical1 : xbsIndex_r4/Logical  logical_function=OR  inputs=2  en=off  latency=0  precision=Full  arith_type=Unsigned  n_bits=16  bin_pt=0  align_bp=on  dbl_ovrd=off  block_type=logical
      settings: block_version=11.4
  Register : xbsIndex_r4/Register  init=0  rst=on  en=on  dbl_ovrd=off  block_type=register
      settings: block_version=11.4
  RegisterX : xbsIndex_r4/Register  init=1  rst=on  en=on  dbl_ovrd=off  block_type=register
      settings: block_version=11.4
  RegisterY : xbsIndex_r4/Register  init=1  rst=on  en=on  dbl_ovrd=off  block_type=register
      settings: block_version=11.4
  RegisterZ : xbsIndex_r4/Register  init=1  rst=on  en=on  dbl_ovrd=off  block_type=register
      settings: block_version=11.4
  posedge : casper_library/Misc/posedge  Tag=Rising Edge Detector  SystemSampleTime=-1
  sync : Outport  OutDataType=sfix(16)  OutScaling=2^0
  X : Outport  Port=2  OutDataType=sfix(16)  OutScaling=2^0
  Y : Outport  Port=3  OutDataType=sfix(16)  OutScaling=2^0
  Z : Outport  Port=4  OutDataType=sfix(16)  OutScaling=2^0
  X_get : Outport  Port=5  OutDataType=sfix(16)  OutScaling=2^0
  Y_get : Outport  Port=6  OutDataType=sfix(16)  OutScaling=2^0
  Z_get : Outport  Port=7  OutDataType=sfix(16)  OutScaling=2^0
  wires:
  DelayZ/1 -> Z/1
  DelayY/1 -> Y/1
  ConstantX/1 -> RegisterX/1
  ConstantY/1 -> RegisterY/1
  ConstantZ/1 -> RegisterZ/1
  syncX/1 -> RegisterX/3
  syncY/1 -> RegisterY/3
  syncZ/1 -> RegisterZ/3
  DelayX/1 -> X/1
  dataX/1 -> DelayX/1
  dataY/1 -> DelayY/1
  dataZ/1 -> DelayZ/1
  RegisterY/1 -> Y_get/1, Logical/2
  RegisterX/1 -> X_get/1, Logical/3
  RegisterZ/1 -> Z_get/1, Logical/1
  Logical/1 -> Register/1, Register/3
  posedge/1 -> Delay/1
  Delay/1 -> sync/1
  Register/1 -> Logical1/1, posedge/1
  rst/1 -> Logical1/2, Register/2
  Logical1/1 -> RegisterX/2, RegisterY/2, RegisterZ/2

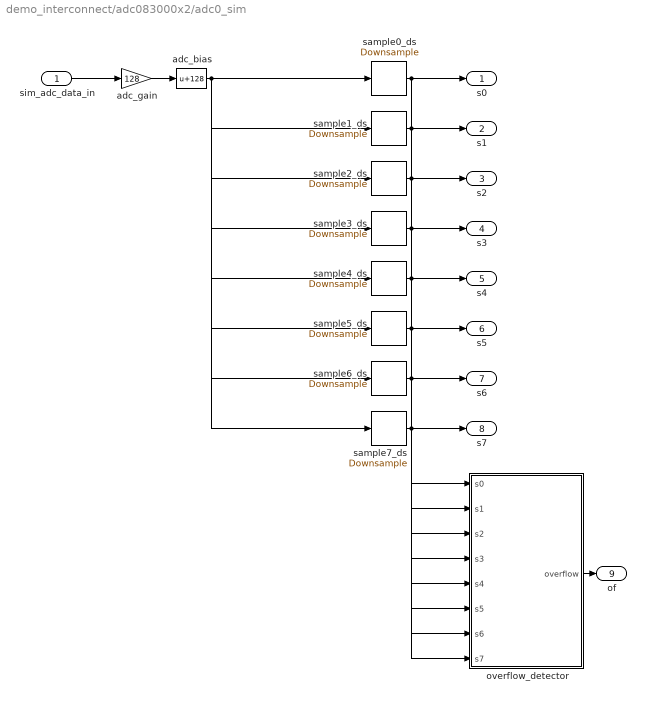
== system demo_interconnect/adc083000x2/adc0_sim ==
  sim_adc_data_in : Inport  OutDataType=sfix(16)  OutScaling=2^0
  adc_bias : Bias  Bias=128  SaturateOnIntegerOverflow=on
  adc_gain : Gain  Gain=128  ParameterDataType=sfix(16)  ParameterScaling=2^0  OutDataType=sfix(16)  OutScaling=2^0
  overflow_detector : Subsystem  AncestorBlock=casper_library/Misc/of_detect_bus  mask(of_detect_bus){nStreams=8, bit_width=8}
      mask prompts: nStreams "Number of Streams"; bit_width "Bit Width"
      mask init:
      | adc_overflow_detector_init(gcb, ...
      |     'nStreams', nStreams, ...
      |     'bit_width', bit_width);
  sample0_ds : dspsigops/Downsample  N=8  phase=1  ic=0  smode=Force single rate  fmode=Maintain input frame size
  sample1_ds : dspsigops/Downsample  N=8  phase=2  ic=0  smode=Force single rate  fmode=Maintain input frame size
  sample2_ds : dspsigops/Downsample  N=8  phase=3  ic=0  smode=Force single rate  fmode=Maintain input frame size
  sample3_ds : dspsigops/Downsample  N=8  phase=4  ic=0  smode=Force single rate  fmode=Maintain input frame size
  sample4_ds : dspsigops/Downsample  N=8  phase=5  ic=0  smode=Force single rate  fmode=Maintain input frame size
  sample5_ds : dspsigops/Downsample  N=8  phase=6  ic=0  smode=Force single rate  fmode=Maintain input frame size
  sample6_ds : dspsigops/Downsample  N=8  phase=7  ic=0  smode=Force single rate  fmode=Maintain input frame size
  sample7_ds : dspsigops/Downsample  N=8  phase=0  ic=0  smode=Force single rate  fmode=Maintain input frame size
  s0 : Outport  OutDataType=sfix(16)  OutScaling=2^0
  s1 : Outport  Port=2  OutDataType=sfix(16)  OutScaling=2^0
  s2 : Outport  Port=3  OutDataType=sfix(16)  OutScaling=2^0
  s3 : Outport  Port=4  OutDataType=sfix(16)  OutScaling=2^0
  s4 : Outport  Port=5  OutDataType=sfix(16)  OutScaling=2^0
  s5 : Outport  Port=6  OutDataType=sfix(16)  OutScaling=2^0
  s6 : Outport  Port=7  OutDataType=sfix(16)  OutScaling=2^0
  s7 : Outport  Port=8  OutDataType=sfix(16)  OutScaling=2^0
  of : Outport  Port=9  OutDataType=sfix(16)  OutScaling=2^0
  wires:
  sim_adc_data_in/1 -> adc_gain/1
  adc_gain/1 -> adc_bias/1
  overflow_detector/1(overflow) -> of/1
  adc_bias/1 -> sample0_ds/1, sample1_ds/1, sample2_ds/1, sample3_ds/1, sample4_ds/1, sample5_ds/1, sample6_ds/1, sample7_ds/1
  sample0_ds/1 -> overflow_detector/1(s0), s0/1
  sample1_ds/1 -> overflow_detector/2(s1), s1/1
  sample2_ds/1 -> overflow_detector/3(s2), s2/1
  sample3_ds/1 -> overflow_detector/4(s3), s3/1
  sample4_ds/1 -> overflow_detector/5(s4), s4/1
  sample5_ds/1 -> overflow_detector/6(s5), s5/1
  sample6_ds/1 -> overflow_detector/7(s6), s6/1
  sample7_ds/1 -> overflow_detector/8(s7), s7/1

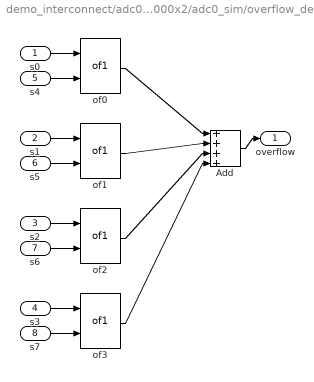
== system demo_interconnect/adc083000x2/adc0_sim/overflow_detector ==
  s0 : Inport  OutDataType=fixdt(1, 16)  OutScaling=2^0
  s1 : Inport  Port=2  OutDataType=fixdt(1, 16)  OutScaling=2^0
  s2 : Inport  Port=3  OutDataType=fixdt(1, 16)  OutScaling=2^0
  s3 : Inport  Port=4  OutDataType=fixdt(1, 16)  OutScaling=2^0
  s4 : Inport  Port=5  OutDataType=fixdt(1, 16)  OutScaling=2^0
  s5 : Inport  Port=6  OutDataType=fixdt(1, 16)  OutScaling=2^0
  s6 : Inport  Port=7  OutDataType=fixdt(1, 16)  OutScaling=2^0
  s7 : Inport  Port=8  OutDataType=fixdt(1, 16)  OutScaling=2^0
  Add : Sum  Inputs=++++  OutDataType=fixdt(1, 16)  OutScaling=2^-10
  of{0..3} (4 alike) : casper_library/Misc/of1  SystemSampleTime=-1  bit_num=0  n_adc_bits=8
  overflow : Outport  OutDataType=fixdt(1, 16)  OutScaling=2^0
  wires:
  s0/1 -> of0/1
  s4/1 -> of0/2
  of0/1 -> Add/1
  s1/1 -> of1/1
  s5/1 -> of1/2
  of1/1 -> Add/2
  s2/1 -> of2/1
  s6/1 -> of2/2
  of2/1 -> Add/3
  s3/1 -> of3/1
  s7/1 -> of3/2
  of3/1 -> Add/4
  Add/1 -> overflow/1
